simulink model "sin_gen"  (Simulink 8.1)
settings: Solver=ode45  StartTime=0.0  StopTime=35e-6  RelTol=1e-3
undefined symbols (not defined in the file): get
libraries: simulink x3, commutil2 x3, commnoisgen2 x1, dspspect3 x1, dspsnks4 x1
settings Model: Creator=Admin  LastModifiedBy=zhuk
settings DebuggingCC: StrictBusMsg=Warning

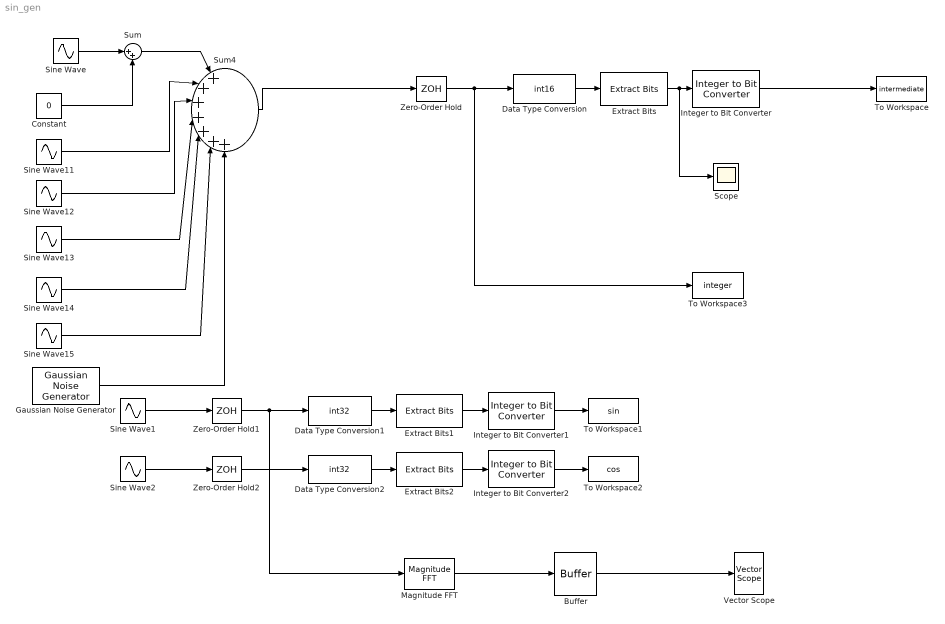
== system sin_gen ==
  Buffer : Buffer  TreatMby1Signals=One channel
  Constant : Constant  Value=0
  Data Type Conversion : DataTypeConversion  OutDataTypeStr=int16
  Data Type Conversion1 : DataTypeConversion  OutDataTypeStr=int32  SampleTime=1/200e6
  Data Type Conversion2 : DataTypeConversion  OutDataTypeStr=int32  SampleTime=1/200e6
  Extract Bits : simulink/Logic and Bit Operations/Extract Bits  bitsToExtract=Range of bits  numBits=8  bitIdxRange=[0 13]  outScalingMode=Preserve fixed-point scaling
  Extract Bits1 : simulink/Logic and Bit Operations/Extract Bits  bitsToExtract=Range of bits  numBits=8  bitIdxRange=[0 15]  outScalingMode=Preserve fixed-point scaling
  Extract Bits2 : simulink/Logic and Bit Operations/Extract Bits  bitsToExtract=Range of bits  numBits=8  bitIdxRange=[0 15]  outScalingMode=Preserve fixed-point scaling
  Gaussian Noise Generator : commnoisgen2/Gaussian Noise Generator  m=0  d=0  s=41  Ts=1/100e6  frameBased=off  sampPerFrame=1  orient=off  outDataType=double
  Integer to Bit Converter : commutil2/Integer to Bit Converter  nbits=14  signedInputValues=Signed  bitOrder=MSB first  outDtype=Inherit via internal rule
  Integer to Bit Converter1 : commutil2/Integer to Bit Converter  nbits=16  signedInputValues=Signed  bitOrder=MSB first  outDtype=Inherit via internal rule
  Integer to Bit Converter2 : commutil2/Integer to Bit Converter  nbits=16  signedInputValues=Signed  bitOrder=MSB first  outDtype=Inherit via internal rule
  Magnitude FFT : dspspect3/Magnitude FFT  mag_or_magsq=Magnitude squared  FFTImplementation=Auto  fftLenInherit=off  fftsize=64
  Scope : Scope
  Sine Wave : Sin  Amplitude=512  Frequency=2*pi*2e6  SampleTime=0
  Sine Wave1 : Sin  Amplitude=15  Frequency=2*pi*10e6  SampleTime=0
  Sine Wave11 : Sin  Amplitude=0  Frequency=2*pi*70e6  Phase=pi  SampleTime=0
  Sine Wave12 : Sin  Amplitude=0  Frequency=2*pi*80e6  Phase=pi/2  SampleTime=0
  Sine Wave13 : Sin  Amplitude=0  Frequency=2*pi*65e6  Phase=pi  SampleTime=0
  Sine Wave14 : Sin  Amplitude=0  Frequency=2*pi*60e6  Phase=pi  SampleTime=0
  Sine Wave15 : Sin  Amplitude=0  Frequency=2*pi*82.4e6  Phase=pi  SampleTime=0
  Sine Wave2 : Sin  Amplitude=15  Frequency=2*pi*20e6  Phase=pi/2  SampleTime=0
  Sum : Sum  Inputs=|++
  Sum4 : Sum  Inputs=|+++++++
  To Workspace : ToWorkspace  VariableName=intermediate  SampleTime=-1
  To Workspace1 : ToWorkspace  VariableName=sin  SampleTime=1/200e6
      settings: MaxDataPoints=100
  To Workspace2 : ToWorkspace  VariableName=cos  SampleTime=1/200e6
      settings: MaxDataPoints=100
  To Workspace3 : ToWorkspace  VariableName=integer  SampleTime=-1
  Vector Scope : dspsnks4/Vector Scope  ScopeProperties=on  Domain=Time  HorizSpan=64  DisplayProperties=off  AxisGrid=on  Memory=off  FrameNumber=on  AxisLegend=off  AxisZoom=off  OpenScopeAtSimStart=on  OpenScopeImmediately=off  FigPos=get(0,'defaultfigureposition')  AxisProperties=off  XUnits=Hertz  XRange=[0...Fs/2]  InheritXIncr=on  XIncr=1  XLabel=Time  XLimit=Auto  XMin=0  XMax=1  XStart=0  YUnits=dB  YLabel=Amplitude  LineProperties=off  XAxisParamsVer=6.9
      settings: YMin=-10  YMax=10
  Zero-Order Hold : ZeroOrderHold  SampleTime=1/50e6
  Zero-Order Hold1 : ZeroOrderHold  SampleTime=1/200e6
  Zero-Order Hold2 : ZeroOrderHold  SampleTime=1/200e6
  wires:
  Sine Wave11/1 -> Sum4/2
  Sine Wave12/1 -> Sum4/3
  Sine Wave13/1 -> Sum4/4
  Zero-Order Hold/1 -> To Workspace3/1, Data Type Conversion/1
  Integer to Bit Converter/1 -> To Workspace/1
  Data Type Conversion/1 -> Extract Bits/1
  Extract Bits/1 -> Scope/1, Integer to Bit Converter/1
  Sum4/1 -> Zero-Order Hold/1
  Sine Wave14/1 -> Sum4/5
  Sine Wave15/1 -> Sum4/6
  Gaussian Noise Generator/1 -> Sum4/7
  Zero-Order Hold1/1 -> Magnitude FFT/1, Data Type Conversion1/1
  Integer to Bit Converter1/1 -> To Workspace1/1
  Data Type Conversion1/1 -> Extract Bits1/1
  Extract Bits1/1 -> Integer to Bit Converter1/1
  Sine Wave1/1 -> Zero-Order Hold1/1
  Zero-Order Hold2/1 -> Data Type Conversion2/1
  Integer to Bit Converter2/1 -> To Workspace2/1
  Data Type Conversion2/1 -> Extract Bits2/1
  Extract Bits2/1 -> Integer to Bit Converter2/1
  Sine Wave2/1 -> Zero-Order Hold2/1
  Sine Wave/1 -> Sum/1
  Sum/1 -> Sum4/1
  Constant/1 -> Sum/2
  Magnitude FFT/1 -> Buffer/1
  Buffer/1 -> Vector Scope/1
